simulink library "csu_ini_initial_conditions_lib"  (R2014b)
settings: Solver=ode45  SolverMode=SingleTasking  StartTime=0.0  StopTime=10.0  RelTol=1e-3
values from neighbouring files (symbols this model uses):
  ini_landed_flag = boolean(0)    [csu_ini_initial_conditions_init.m]
undefined symbols (not defined in the file or in its folder): sim_time_step_size
undefined symbols (not defined in the file): ini_position_v
libraries: util_common_lib x3, simulink x1, util_info_lib x1
settings Model: ExtModeAutoUpdateStatusClock=off  Creator=daniloviazzo  LastModifiedBy=mstewart

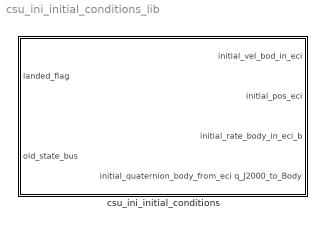
== system csu_ini_initial_conditions_lib ==
  csu_ini_initial_conditions : Subsystem

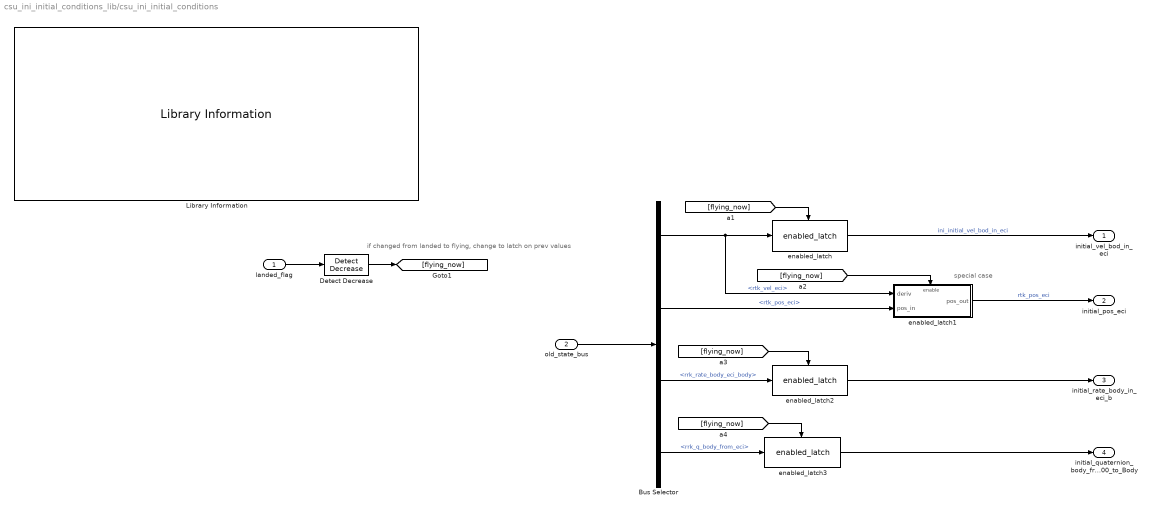
== system csu_ini_initial_conditions_lib/csu_ini_initial_conditions ==
  note: if changed from landed to flying, change to latch on prev values
  note: special case
  landed_flag : Inport
  old_state_bus : Inport  Port=2
  Bus Selector : BusSelector  OutputSignals=rtk_vel_eci,rtk_pos_eci,rrk_rate_body_eci_body,rrk_q_body_from_eci
  Detect Decrease : simulink/Logic and Bit Operations/Detect Decrease  vinit=ini_landed_flag  InputProcessing=Inherited  OutDataTypeStr=boolean
  Library Information : util_info_lib/Library Information  owner='NONE'
  enabled_latch : util_common_lib/enabled_latch  initial_output=ini_velocity_v
  enabled_latch1 : Subsystem  mask{initial_output=ini_position_v}
      mask prompts: initial_output "Initial Output Value"
  enabled_latch2 : util_common_lib/enabled_latch  initial_output=ini_rate_v
  enabled_latch3 : util_common_lib/enabled_latch  initial_output=ini_quaternion_v
  initial_vel_bod_in_eci : Outport
  initial_pos_eci : Outport  Port=2
  initial_rate_body_in_eci_b : Outport  Port=3
  initial_quaternion_body_from_eci q_J2000_to_Body : Outport  Port=4
  wires:
  enabled_latch3/1 -> initial_quaternion_body_from_eci q_J2000_to_Body/1
  enabled_latch2/1 -> initial_rate_body_in_eci_b/1
  enabled_latch1/1(pos_out) -> initial_pos_eci/1  "rtk_pos_eci"
  [flying_now] -> enabled_latch3/Enable
  [flying_now] -> enabled_latch2/Enable
  Bus Selector/4 -> enabled_latch3/1  "<rrk_q_body_from_eci>"
  Bus Selector/3 -> enabled_latch2/1  "<rrk_rate_body_eci_body>"
  [flying_now] -> enabled_latch1/Enable
  Bus Selector/2 -> enabled_latch1/2(pos_in)  "<rtk_pos_eci>"
  Bus Selector/1 -> enabled_latch/1, enabled_latch1/1(deriv)  "<rtk_vel_eci>"
  [flying_now] -> enabled_latch/Enable
  Detect Decrease/1 -> [flying_now]
  landed_flag/1 -> Detect Decrease/1
  old_state_bus/1 -> Bus Selector/1
  enabled_latch/1 -> initial_vel_bod_in_eci/1  "ini_initial_vel_bod_in_eci"

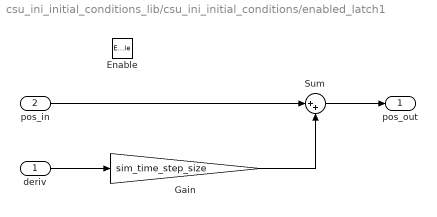
== system csu_ini_initial_conditions_lib/csu_ini_initial_conditions/enabled_latch1 ==
  deriv : Inport
  pos_in : Inport  Port=2
  Enable : EnablePort
  Gain : Gain  Gain=sim_time_step_size
  Sum : Sum  Inputs=|++
  pos_out : Outport  InitialOutput=initial_output
  wires:
  Gain/1 -> Sum/2
  deriv/1 -> Gain/1
  Sum/1 -> pos_out/1
  pos_in/1 -> Sum/1
